simulink model "Final_System_Model_V10"  (R2018a)
settings: Solver=VariableStepAuto  StartTime=0  StopTime=250  FixedStep=0.5  RelTol=1e-3
PreLoadFcn:
  | Ts_Power=1e-6;
  | Ts_Control=100e-6;
undefined symbols (not defined in the file): DiscIntNeverNeededParam, sigbuilder_block
libraries: simulink x24, fl_lib x16, powerlib x15, nesl_utility x8, powerlib_meascontrol x5, re_lib x1
(part 6 of 8)

== system Final_System_Model_V10/Full System/Subsystem1/80KW Fuel Cell Stack_1/Load ==
  note: This Block models the Load Profile as dictated by the ship Resistance in the River Nile
  Signal : Inport
  Bus Selector : BusSelector  OutputSignals=Cell Output Voltage (V),Number Of Cells
  Current from Load profile of one day : Subsystem  Tag=STV Subsys  LoadFcn=sigbuilder_block('load');  StartFcn=sigbuilder_block('start');  StopFcn=sigbuilder_block('stop');  ClipboardFcn=sigbuilder_block('clipboard');  mask(Sigbuilder block){tuvar=[0:10]}
      mask help: Simulink:masks:SigbuilderBlock_MD
      mask init:
      | if ~strcmp(get_param(bdroot(gcbh),'SimulationStatus'),'stopped') tuvar = sigbuilder_block('maskInit'); end
      settings: CopyFcn=sigbuilder_block('copy');  DeleteFcn=sigbuilder_block('delete');  ModelCloseFcn=sigbuilder_block('modelClose');  PreSaveFcn=sigbuilder_block('preSave');  PauseFcn=sigbuilder_block('pause');  ContinueFcn=sigbuilder_block('continue');  NameChangeFcn=sigbuilder_block('namechange');  OpenFcn=sigbuilder_block('open',[403.5 117 550.5 359.25 ]);  CloseFcn=sigbuilder_block('close');
      mask Display: plot(0, 0, 100, 100,[2, 2, 32, 32, 2], [68, 8, 8, 68, 68],[32, 2], [38, 38], [32, 19, 2],[53, 60, 44], [32, 17, 17, 2],[16, 16, 31, 31]);txt = getActiveGroup(gcbh);text(2, 100, txt,'verticalAlignment', 'top');
  Product : Product
  Terminator : Terminator
  Terminator1 : Terminator
  Total Output Voltage (V) : Outport
  wires:
  Current from Load profile of one day/1(Signal 1) -> Terminator/1  "Current from Load profile (Alex to Aswan)"
  Bus Selector/2 -> Product/2  "<Number Of Cells>"
  Current from Load profile of one day/2(Signal 2) -> Terminator1/1  "Current from Load profile (Alex to Aswan)"
  Product/1 -> Total Output Voltage (V)/1  "Total Output Voltage (V)"
  Bus Selector/1 -> Product/1  "<Cell Output Voltage (V)>"
  Signal/1 -> Bus Selector/1

== system Final_System_Model_V10/Full System/Subsystem3/DC-DC converter1/Subsystem ==
  duty cycle : Inport
  I in : Inport  Port=2
  V in : Inport  Port=3
  Constant : Constant
  I out : Product  Inputs=*/
  Multiply : Product
  Multiply1 : Product
  Subtract : Sum  Inputs=+-
  V out : Product  Inputs=*/
  efficiency : Gain  Gain=0.98
  efficiency1 : Gain  Gain=0.98
  I o : Outport
  V o : Outport  Port=2
  wires:
  V in/1 -> efficiency1/1
  I out/1 -> I o/1
  V out/1 -> V o/1
  I in/1 -> efficiency/1
  efficiency1/1 -> Multiply1/1
  Multiply1/1 -> V out/1
  duty cycle/1 -> Multiply1/2, I out/2, Subtract/2
  Constant/1 -> Subtract/1
  Multiply/1 -> I out/1
  efficiency/1 -> Multiply/2
  Subtract/1 -> V out/2, Multiply/1

== system Final_System_Model_V10/Full System/Subsystem3/DC-DC converter1/duty cycle ==
  V in : Inport
  V req : Inport  Port=2
  Add : Sum
  Constant : Constant
  Divide : Product  Inputs=*/
  Gain : Gain  Gain=0.98
  Subtract : Sum  Inputs=+-
  tag scope: duty_cycle_battery=global
  wires:
  Divide/1 -> Subtract/2
  Gain/1 -> Add/1, Divide/1
  Add/1 -> Divide/2
  Constant/1 -> Subtract/1
  V in/1 -> Gain/1
  V req/1 -> Add/2
  Subtract/1 -> [duty_cycle_battery]

== system Final_System_Model_V10/Full System/Subsystem3/Subsystem/1st Mode ==
  delta : Inport
  Fuel Cells Output (KW) : Inport  Port=2
  Add : Sum  Inputs=+-
  Compare To Constant : simulink/Logic and Bit Operations/Compare To Constant  relop=>=  const=0  OutDataTypeStr=boolean
  Compare To Constant1 : simulink/Logic and Bit Operations/Compare To Constant  relop=<  const=72  OutDataTypeStr=boolean
  Logical Operator : Logic  AllPortsSameDT=off  OutDataTypeStr=boolean
  Switch15 : Switch  Criteria=u2 > Threshold
  Zero : Constant  Value=0
  Load to battery (KW) : Outport
  wires:
  Compare To Constant1/1 -> Logical Operator/2
  Compare To Constant/1 -> Logical Operator/1
  Zero/1 -> Switch15/3
  delta/1 -> Compare To Constant1/1, Add/1, Compare To Constant/1
  Switch15/1 -> Load to battery (KW)/1
  Logical Operator/1 -> Switch15/2
  Fuel Cells Output (KW)/1 -> Add/2
  Add/1 -> Switch15/1

== system Final_System_Model_V10/Full System/Subsystem3/Subsystem/2nd Mode ==
  delta : Inport
  Fuel Cells Output (KW) : Inport  Port=2
  Add : Sum  Inputs=+-
  Compare To Constant : simulink/Logic and Bit Operations/Compare To Constant  relop=>=  const=88  OutDataTypeStr=boolean
  Compare To Constant1 : simulink/Logic and Bit Operations/Compare To Constant  relop=<=  const=90  OutDataTypeStr=boolean
  Logical Operator : Logic  AllPortsSameDT=off  OutDataTypeStr=boolean
  Switch15 : Switch  Criteria=u2 > Threshold
  Zero : Constant  Value=0
  Battery to load (KW) : Outport
  wires:
  Switch15/1 -> Battery to load (KW)/1
  Fuel Cells Output (KW)/1 -> Add/2
  Compare To Constant1/1 -> Logical Operator/2
  Logical Operator/1 -> Switch15/2
  Compare To Constant/1 -> Logical Operator/1
  delta/1 -> Compare To Constant1/1, Compare To Constant/1, Add/1
  Zero/1 -> Switch15/3
  Add/1 -> Switch15/1

== system Final_System_Model_V10/Full System/Subsystem3/Subsystem/5th Mode ==
  delta : Inport
  Fuel Cells Output (KW) : Inport  Port=2
  Add : Sum  Inputs=+-
  Compare To Constant : simulink/Logic and Bit Operations/Compare To Constant  relop=>=  const=110  OutDataTypeStr=boolean
  Compare To Constant1 : simulink/Logic and Bit Operations/Compare To Constant  relop=<=  const=162  OutDataTypeStr=boolean
  Logical Operator : Logic  AllPortsSameDT=off  OutDataTypeStr=boolean
  Switch15 : Switch  Criteria=u2 > Threshold
  Zero : Constant  Value=0
  Battery to load (KW) : Outport
  wires:
  Add/1 -> Switch15/1
  Zero/1 -> Switch15/3
  delta/1 -> Add/1, Compare To Constant/1, Compare To Constant1/1
  Compare To Constant/1 -> Logical Operator/1
  Logical Operator/1 -> Switch15/2
  Compare To Constant1/1 -> Logical Operator/2
  Fuel Cells Output (KW)/1 -> Add/2
  Switch15/1 -> Battery to load (KW)/1

== system Final_System_Model_V10/Full System/Subsystem3/Subsystem/7th Mode ==
  delta : Inport
  Fuel Cells Output (KW) : Inport  Port=2
  Add : Sum  Inputs=+-
  Compare To Constant : simulink/Logic and Bit Operations/Compare To Constant  relop=>=  const=198  OutDataTypeStr=boolean
  Compare To Constant1 : simulink/Logic and Bit Operations/Compare To Constant  relop=<=  const=214  OutDataTypeStr=boolean
  Logical Operator : Logic  AllPortsSameDT=off  OutDataTypeStr=boolean
  Switch15 : Switch  Criteria=u2 > Threshold
  Zero : Constant  Value=0
  Battery to load (KW) : Outport
  wires:
  Switch15/1 -> Battery to load (KW)/1
  Fuel Cells Output (KW)/1 -> Add/2
  Compare To Constant1/1 -> Logical Operator/2
  Logical Operator/1 -> Switch15/2
  Compare To Constant/1 -> Logical Operator/1
  delta/1 -> Compare To Constant1/1, Compare To Constant/1, Add/1
  Zero/1 -> Switch15/3
  Add/1 -> Switch15/1

== system Final_System_Model_V10/Full System/Electrolysers/260 KW Electrolyzer Stack_1/electrolyser stack/electrolyser cell ==
  In1 : Inport
  In2 : Inport  Port=2
  In3 : Inport  Port=3
  (1/T)/(1/T_ref) : Subsystem
  Constant2 : Constant  Value=1/298
  Eta_B : Subsystem
  F : Constant  Value=96485.33289
  H2 flow rate : Subsystem
  R : Constant  Value=8.314
  Sum : Sum  Inputs=4
  V_0 : Subsystem
  eta_a : Subsystem
  eta_c : Subsystem
  Out1 : Outport
  Out2 : Outport  Port=2
  wires:
  eta_c/1(Out1) -> Sum/4
  In2/1 -> H2 flow rate/1(In1), eta_c/4(In4), eta_a/3(In3), Eta_B/3(In3)
  R/1 -> eta_a/2(In2), eta_a/4(In4), eta_c/2(In2), Eta_B/1(In1)
  In1/1 -> eta_a/5(In5), eta_c/3(In3), Eta_B/2(In2), (1/T)/(1/T_ref)/1(In1), V_0/1(In1)
  (1/T)/(1/T_ref)/1(Out1) -> eta_a/1(In1), eta_c/1(In1)
  eta_a/1(Out1) -> Sum/3
  Constant2/1 -> Eta_B/4(In4), (1/T)/(1/T_ref)/2(In2)
  Eta_B/1(Out1) -> Sum/2
  F/1 -> eta_a/6(In6), eta_c/5(In5), H2 flow rate/2(In2)
  V_0/1(Out1) -> Sum/1
  Sum/1 -> Out1/1
  In3/1 -> H2 flow rate/3(In3)
  H2 flow rate/1(Out1) -> Out2/1

== system Final_System_Model_V10/Full System/Electrolysers/93 KW Electrolyzer Stack_2/electrolyser stack/electrolyser cell ==
  In1 : Inport
  In2 : Inport  Port=2
  In3 : Inport  Port=3
  (1/T)/(1/T_ref) : Subsystem
  Constant2 : Constant  Value=1/298
  Eta_B : Subsystem
  F : Constant  Value=96485.33289
  H2 flow rate : Subsystem
  R : Constant  Value=8.314
  Sum : Sum  Inputs=4
  V_0 : Subsystem
  eta_a : Subsystem
  eta_c : Subsystem
  Out1 : Outport
  Out2 : Outport  Port=2
  wires:
  H2 flow rate/1(Out1) -> Out2/1
  In3/1 -> H2 flow rate/3(In3)
  Sum/1 -> Out1/1
  V_0/1(Out1) -> Sum/1
  F/1 -> H2 flow rate/2(In2), eta_c/5(In5), eta_a/6(In6)
  Eta_B/1(Out1) -> Sum/2
  Constant2/1 -> (1/T)/(1/T_ref)/2(In2), Eta_B/4(In4)
  eta_a/1(Out1) -> Sum/3
  (1/T)/(1/T_ref)/1(Out1) -> eta_c/1(In1), eta_a/1(In1)
  In1/1 -> V_0/1(In1), (1/T)/(1/T_ref)/1(In1), Eta_B/2(In2), eta_c/3(In3), eta_a/5(In5)
  R/1 -> Eta_B/1(In1), eta_c/2(In2), eta_a/4(In4), eta_a/2(In2)
  In2/1 -> Eta_B/3(In3), eta_a/3(In3), eta_c/4(In4), H2 flow rate/1(In1)
  eta_c/1(Out1) -> Sum/4

== system Final_System_Model_V10/Full System/Solar Panel + Solar Charge Controller/PV Insert inputs here/Subsystem/C to K Converter  ==
  T_o : Inport
  Sum : Sum  Inputs=|++
  Sum1 : Sum  Inputs=|++
  T_ref : Constant  Value=25
  constant : Constant  Value=273.12
  T_ak : Outport
  T_rk : Outport  Port=2
  wires:
  constant/1 -> Sum1/1, Sum/2
  T_o/1 -> Sum/1  "T_act (c)"
  T_ref/1 -> Sum1/2  "T_ref (c)"
  Sum/1 -> T_ak/1  "T_act(k)"
  Sum1/1 -> T_rk/1  "T_ref(k)"

== system Final_System_Model_V10/Full System/Solar Panel + Solar Charge Controller/PV Insert inputs here/Subsystem/I o ==
  T_ak : Inport
  T_rk : Inport  Port=2
  I_on : Inport  Port=3
  Constant : Constant
  Electron charge : Constant  Value=1.6*10^(-19)
  Exp(fn(1)) : Fcn  Expr=exp(u(1))
  Fcn : Fcn  Expr=(u(1))^3
  Product : Product  Inputs=/***/
  Product1 : Product  Inputs=*/
  Product2 : Product  Inputs=*/
  Product3 : Product  Inputs=*/
  Product4 : Product  Inputs=3
  Sum : Sum  Inputs=|+-
  band gap energy (Eg) : Constant  Value=1.1
  boltzamann constant : Constant  Value=1.3805*10^(-23)
  ideality factor depend on material : Constant  Value=1.14
  I_o : Outport
  wires:
  Electron charge/1 -> Product/2  "e"
  boltzamann constant/1 -> Product/1  "k"
  Product2/1 -> Sum/2  "1/T"
  I_on/1 -> Product4/3  "I_on"
  band gap energy (Eg)/1 -> Product/3  "Eg"
  Sum/1 -> Product/4  "((1/Tn)-(1/T))"
  Product3/1 -> Fcn/1  "T/Tn"
  Product1/1 -> Sum/1  "1/Tn"
  Constant/1 -> Product2/1, Product1/1
  ideality factor depend on material/1 -> Product/5  "a"
  T_ak/1 -> Product3/1, Product2/2
  Fcn/1 -> Product4/2  "(T/Tn)^3"
  Product/1 -> Exp(fn(1))/1  "Fn(1)"
  Exp(fn(1))/1 -> Product4/1  "Exp(fn(1))"
  T_rk/1 -> Product1/2, Product3/2
  Product4/1 -> I_o/1

== system Final_System_Model_V10/Full System/Solar Panel + Solar Charge Controller/PV Insert inputs here/Subsystem/I on ==
  T_ref : Inport
  I_scn : Inport  Port=2
  Num series : Inport  Port=3
  V_oc : Inport  Port=4
  Electron charge : Constant  Value=1.6*10^(-19)
  Fcn : Fcn  Expr=(u(1))/(exp(u(2))-u(1))
  Mux : Mux  Inputs=3
  Product : Product  Inputs=//**//
  boltzamann constant : Constant  Value=1.3805*10^(-23)
  constant : Constant
  ideality factor : Constant  Value=1.1415
  I_on : Outport
  wires:
  Num series/1 -> Product/1  "num_series_cells"
  boltzamann constant/1 -> Product/2  "K"
  Electron charge/1 -> Product/3  "q"
  ideality factor/1 -> Product/5  "a"
  T_ref/1 -> Product/6  "T_ref(k)"
  Product/1 -> Mux/2
  I_scn/1 -> Mux/1
  constant/1 -> Mux/3
  Mux/1 -> Fcn/1
  Fcn/1 -> I_on/1
  V_oc/1 -> Product/4

== system Final_System_Model_V10/Full System/Solar Panel + Solar Charge Controller/PV Insert inputs here/Subsystem/I ph due to radiation  ==
  insolation : Inport
  T_ak : Inport  Port=2
  T_rk : Inport  Port=3
  I_scn : Inport  Port=4
  Product : Product
  Product1 : Product
  SC_temp COFF const : Constant  Value=0.0017
  Sum : Sum  Inputs=|++
  Sum1 : Sum  Inputs=|+-
  I_photon : Outport
  wires:
  Product/1 -> I_photon/1  "photons current"
  insolation/1 -> Product/1
  T_ak/1 -> Sum1/1  "actual temp(k)"
  T_rk/1 -> Sum1/2  "referance temp(k)"
  Sum/1 -> Product/2
  I_scn/1 -> Sum/2  "nominal short circuit current"
  Product1/1 -> Sum/1
  SC_temp COFF const/1 -> Product1/1
  Sum1/1 -> Product1/2

== system Final_System_Model_V10/Full System/Solar Panel + Solar Charge Controller/PV Insert inputs here/Subsystem/I pv ==
  V_PV : Inport
  I_photon : Inport  Port=2
  I_o : Inport  Port=3
  Ns*A*Kt1 : Inport  Port=4
  Rp Shunt resistance : Inport  Port=5
  Electron charge : Constant  Value=1.6*10^(-19)
  IPV = u(3)-u(4)*(exp((u(2)*(u(1)+u(6)))/(u(5)))-1) : Fcn  Expr=u(3)-u(4)*(exp((u(2)*(u(1)+u(6)))/(u(5)))-1)-u(7)
  Mux : Mux  Inputs=7
  Product : Product  Inputs=*/
  Rs : Gain  Gain=.4
  Sum : Sum  Inputs=|++
  I_PV : Outport
  wires:
  IPV = u(3)-u(4)*(exp((u(2)*(u(1)+u(6)))/(u(5)))-1)/1 -> I_PV/1, Rs/1  "I_PV"
  Ns*A*Kt1/1 -> Mux/5
  Mux/1 -> IPV = u(3)-u(4)*(exp((u(2)*(u(1)+u(6)))/(u(5)))-1)/1
  I_o/1 -> Mux/4  "I_o"
  Rs/1 -> Sum/2, Mux/6  "I_PV*Rs"
  Electron charge/1 -> Mux/2  "q"
  I_photon/1 -> Mux/3  "I_ph"
  V_PV/1 -> Sum/1, Mux/1  "V_PV"
  Sum/1 -> Product/1
  Rp Shunt resistance/1 -> Product/2  "Shunt resistance"
  Product/1 -> Mux/7

== system Final_System_Model_V10/Full System/Solar Panel + Solar Charge Controller/PV Insert inputs here/Subsystem/NsAKt Thermal voltafe ==
  T_ak T in kelven : Inport
  N_series series cells : Constant  Value=96
  Product4 : Product  Inputs=4
  boltzamann constant : Constant  Value=1.3805*10^(-23)
  ideality factor depend on material : Constant  Value=1.17
  Ns*a*Kt : Outport
  wires:
  Product4/1 -> Ns*a*Kt/1
  boltzamann constant/1 -> Product4/2
  ideality factor depend on material/1 -> Product4/3
  T_ak T in kelven/1 -> Product4/1
  N_series series cells/1 -> Product4/4

== system Final_System_Model_V10/Full System/Solar Panel + Solar Charge Controller/Solar Charge Controller/MPPT Controller using  "Incremental Conductance + Integral Regulator "  technique /MPPT ==
  note: Maximum power point tracking by incremental conductance method
      | --------------------------------------------------------------
      | Maximum power point is obtained when dP/dV=0  where P= V*I
      | -> d(V*I)/dV = I + V*dI/dV = 0
      | -> dI/dV = -I/V
      |
      | dI, dV  = fundamental components of I and V ripples measured with a sliding time window T_MPPT
      | I , V   = mean values of V and I measured with a sliding time window T_MPPT
      |
      | The integral regulator minimizes the error (dI/dV + I/V)
      | Regulator output = Duty cycle correction
  V_PV : Inport
  I_PV : Inport  Port=2
  on/off : Inport  Port=3
  Add : Sum  Inputs=+-
  Add1 : Sum
  Constant : Constant  Value=0
  Constant1 : Constant  Value=0
  Dead Zone : DeadZone  LowerValue=-0.05  UpperValue=0.05  SaturateOnIntegerOverflow=on
  Discrete-Time Integrator : DiscreteIntegrator  SampleTime=Ts_Control  LimitOutput=on  UpperSaturationLimit=1  LowerSaturationLimit=-1  ICPrevOutput=DiscIntNeverNeededParam  ICPrevScaledInput=DiscIntNeverNeededParam
  Fourier : powerlib_meascontrol/Measurements/Fourier  Freq=1/T_MPPT  n=1  InInit=[0, 0]  Ts=Ts_Control
      settings: SourceProductName=Simscape Power Systems
  Fourier1 : powerlib_meascontrol/Measurements/Fourier  Freq=1/T_MPPT  n=1  InInit=[0, 0]  Ts=Ts_Control
      settings: SourceProductName=Simscape Power Systems
  MPPT Gain : Gain  Gain=5
  Mean : powerlib_meascontrol/Measurements/Mean  Freq=1/T_MPPT  Vinit=0  Ts=Ts_Control
  Mean1 : powerlib_meascontrol/Measurements/Mean  Freq=1/T_MPPT  Vinit=0  Ts=Ts_Control
  Saturation : Saturate  UpperLimit=inf  LowerLimit=eps
  Saturation1 : Saturate  UpperLimit=inf  LowerLimit=eps
  Switch : Switch  Threshold=0.5
  Switch1 : Switch  Threshold=0.5
  Trigonometric Function : Trigonometry  Operator=cos
  deg2rad : Gain  Gain=pi/180
  div : Product  Inputs=*/  RndMeth=Zero
  div1 : Product  Inputs=**  RndMeth=Zero
  div2 : Product  Inputs=*/  RndMeth=Zero
  Delta_D : Outport
  wires:
  Dead Zone/1 -> MPPT Gain/1
  Switch/1 -> Dead Zone/1  "error"
  Saturation1/1 -> div/2
  Saturation/1 -> div2/2
  Switch1/1 -> Delta_D/1
  on/off/1 -> Switch/2, Switch1/2
  Constant1/1 -> Switch1/3
  Discrete-Time Integrator/1 -> Switch1/1  "Delta_D"
  Constant/1 -> Switch/3
  MPPT Gain/1 -> Discrete-Time Integrator/1
  Add1/1 -> Switch/1  "error"
  div2/1 -> Add1/2  "I/V"
  Mean1/1 -> Saturation/1
  Mean/1 -> div2/1
  div1/1 -> Add1/1  "dI/dV"
  Trigonometric Function/1 -> div1/2
  div/1 -> div1/1
  deg2rad/1 -> Trigonometric Function/1
  Add/1 -> deg2rad/1
  Fourier1/1 -> Saturation1/1
  Fourier1/2 -> Add/2
  Fourier/2 -> Add/1
  V_PV/1 -> Mean1/1, Fourier1/1
  I_PV/1 -> Mean/1, Fourier/1
  Fourier/1 -> div/1

== system Final_System_Model_V10/Full System/Solar Panel + Solar Charge Controller/Solar Charge Controller MPPT it is a device which track a point which has the max power/MPPT /P&O  ==
  I_pv : Inport
  V_PV : Inport  Port=2
  P & O : Subsystem
  Saturation : Saturate  UpperLimit=1
  Subsystem1 : Subsystem
  Signal : Outport
  wires:
  P & O/1(signal) -> Saturation/1
  V_PV/1 -> P & O/2(Vpv)
  Saturation/1 -> Subsystem1/1(In1)
  Subsystem1/1(Out1) -> Signal/1
  I_pv/1 -> P & O/1(Ipv)

== system Final_System_Model_V10/Full System/Subsystem1/100KW Fuel Cell Stack_2/From Load Current and Fuel Cell Output Current (A) to Valve Restriction Area (m^2)/Subsystem ==
  In1 : Inport
  Add1 : Sum  Inputs=4
  Bus Creator1 : BusCreator  Inputs=7
  Bus Selector1 : BusSelector  OutputSignals=Output Current (A),3,3:0735e-14,Output Current (A),2,-5:0428e-11,Output Current (A),4:1772e-08,2:7105e-07
  Constant10 : Constant  Value=4.1772e-08
  Constant11 : Constant  Value=2.7105e-07
  Constant6 : Constant  Value=3
  Constant7 : Constant  Value=3.0735e-14
  Constant8 : Constant  Value=2
  Constant9 : Constant  Value=-5.0428e-11
  Math Function2 : Math  Operator=pow  SaturateOnIntegerOverflow=on
  Math Function3 : Math  Operator=pow  SaturateOnIntegerOverflow=on
  Product3 : Product
  Product4 : Product
  Product5 : Product
  Unit Delay3 : UnitDelay  SampleTime=-1
  Valve Opening from Output Current : Outport
  wires:
  Product3/1 -> Add1/1
  Constant9/1 -> Bus Creator1/5  "-5:0428e-11"
  Constant11/1 -> Bus Creator1/7  "2:7105e-07"
  Constant8/1 -> Bus Creator1/4  "2"
  Constant6/1 -> Bus Creator1/2  "3"
  Bus Selector1/5 -> Math Function3/2  "<2>"
  Constant10/1 -> Bus Creator1/6  "4:1772e-08"
  In1/1 -> Unit Delay3/1
  Math Function2/1 -> Product3/1
  Math Function3/1 -> Product4/1
  Bus Selector1/3 -> Product3/2  "<3:0735e-14>"
  Bus Selector1/9 -> Add1/4  "<2:7105e-07>"
  Bus Selector1/2 -> Math Function2/2  "<3>"
  Bus Creator1/1 -> Bus Selector1/1
  Bus Selector1/6 -> Product4/2  "<-5:0428e-11>"
  Bus Selector1/8 -> Product5/2  "<4:1772e-08>"
  Bus Selector1/4 -> Math Function3/1  "<Output Current (A)>"
  Product4/1 -> Add1/2
  Product5/1 -> Add1/3
  Constant7/1 -> Bus Creator1/3  "3:0735e-14"
  Unit Delay3/1 -> Bus Creator1/1  "Output Current (A)"
  Bus Selector1/7 -> Product5/1  "<Output Current (A)>"
  Bus Selector1/1 -> Math Function2/1  "<Output Current (A)>"
  Add1/1 -> Valve Opening from Output Current/1  "Valve Opening from Output Current"

== system Final_System_Model_V10/Full System/Subsystem1/100KW Fuel Cell Stack_2/From Load Current and Fuel Cell Output Current (A) to Valve Restriction Area (m^2)/Subsystem1 ==
  In1 : Inport
  Add : Sum  Inputs=4
  Bus Creator : BusCreator  Inputs=7
  Bus Selector : BusSelector  OutputSignals=|
      | Load Profile Current (A).Required Current
      | (A),3,3:0735e-14,Load Profile Current (A).Required Current
      | (A),2,-5:0428e-11,Load Profile Current (A).Required Current
      | (A),4:1772e-08,2:7105e-07
  Constant : Constant  Value=3
  Constant1 : Constant  Value=3.0735e-14
  Constant2 : Constant  Value=2
  Constant3 : Constant  Value=-5.0428e-11
  Constant4 : Constant  Value=4.1772e-08
  Constant5 : Constant  Value=2.7105e-07
  Math Function : Math  Operator=pow  SaturateOnIntegerOverflow=on
  Math Function1 : Math  Operator=pow  SaturateOnIntegerOverflow=on
  Product : Product
  Product1 : Product
  Product2 : Product
  Unit Delay2 : UnitDelay  SampleTime=-1
  Out1 : Outport
  wires:
  Bus Selector/2 -> Math Function/2  "<3>"
  Bus Selector/5 -> Math Function1/2  "<2>"
  Product/1 -> Add/1
  Constant/1 -> Bus Creator/2  "3"
  Unit Delay2/1 -> Bus Creator/1  "Load Profile Current (A)"
  Constant5/1 -> Bus Creator/7  "2:7105e-07"
  Constant2/1 -> Bus Creator/4  "2"
  Bus Selector/1 -> Math Function/1  "<Required Current (A)>"
  Constant3/1 -> Bus Creator/5  "-5:0428e-11"
  Constant4/1 -> Bus Creator/6  "4:1772e-08"
  Bus Selector/7 -> Product2/1  "<Required Current (A)>"
  Math Function1/1 -> Product1/1
  Bus Selector/9 -> Add/4  "<2:7105e-07>"
  Bus Selector/8 -> Product2/2  "<4:1772e-08>"
  Bus Selector/6 -> Product1/2  "<-5:0428e-11>"
  Constant1/1 -> Bus Creator/3  "3:0735e-14"
  Product1/1 -> Add/2
  Math Function/1 -> Product/1
  Bus Creator/1 -> Bus Selector/1
  Product2/1 -> Add/3
  Bus Selector/3 -> Product/2  "<3:0735e-14>"
  Bus Selector/4 -> Math Function1/1  "<Required Current (A)>"
  In1/1 -> Unit Delay2/1
  Add/1 -> Out1/1

== system Final_System_Model_V10/Full System/Subsystem1/100KW Fuel Cell Stack_2/Fuel Cell Model/ From Current Density (A//cm^2) To Overvoltages (V) ==
  note: This Block calculates all the Resistances in the Fuel Cell
      | 1-Activation Overvoltage 2- Ohmic Overvoltage 3-Concentration Overvoltage
      | INPUTS: INPUTS: A) Current Density (A/cm^2) INPUTS: A) Current Density (A/cm^2)
      | A) Current Density (A/cm^2) OUTPUTS: A) Ohmic Overvoltage (V) OUTPUTS: A) Concentration Overvoltage (V)
      | B) Temperature (c)
      |
      | OUTPUTS:
      | A) Activation Overvoltage (V)
  Current Density (A/cm^2) : Inport
  Temperature (C) : Inport  Port=2
  Activation Overvoltage : Subsystem
  Concentration Overvoltage : Subsystem
  Ohmic Overvoltage : Subsystem
  Activation Overvoltage (V) : Outport
  Ohmic Overvoltage (V) : Outport  Port=2
  Concentration Overvoltage (V) : Outport  Port=3
  Exchange Current Density (i_0) : Outport  Port=4
  wires:
  Temperature (C)/1 -> Activation Overvoltage/1(Temperature/C1)
  Current Density (A/cm^2)/1 -> Activation Overvoltage/2(Current Density (i)(A/cm^2)), Concentration Overvoltage/1(Current Density (i)1), Ohmic Overvoltage/1(Current Density (i ))
  Ohmic Overvoltage/1(V_Resistive) -> Ohmic Overvoltage (V)/1
  Activation Overvoltage/1(Activation Overvoltage1 (V)) -> Activation Overvoltage (V)/1
  Concentration Overvoltage/1("Concentration Overvoltage1 (V) ") -> Concentration Overvoltage (V)/1
  Activation Overvoltage/2(Exchange Current Density (i_0)) -> Exchange Current Density (i_0)/1

== system Final_System_Model_V10/Full System/Subsystem1/100KW Fuel Cell Stack_2/Fuel Cell Model/Air Flow Rate To Current (A) ==
  note: The function of this block is: To calculate the Air Mass Flow Rate in (kg/s) using the Input Current Density (A/cm^2)
      | Inputs: Outputs:
      | a) Current DEnsity (A/cm^2) A) Air Mass Flow Rate (kg/s)
      | b) Cell Area (cm^2)
      | c) Number of Cells
  Current Density (A/cm^2) : Inport
  Cell Area (cm^2) : Inport  Port=2
  Number Of Cells : Inport  Port=3
  Air Molar Mass (Kg) : Constant  Value=28.9647e-3
  Current (A) : Product
  Divide : Product  Inputs=*/
  From Stack Current (A) To Oxygen Mass Flow Rate(kg/s) : Subsystem
  Oxygen Molar Mass per One Mole of Air (Kg) : Constant  Value=6.72e-3
  Product : Product
  Air Mass Flow Rate (kg/s) : Outport
  wires:
  Current (A)/1 -> From Stack Current (A) To Oxygen Mass Flow Rate(kg/s)/1(Current (A))
  Number Of Cells/1 -> From Stack Current (A) To Oxygen Mass Flow Rate(kg/s)/2(Number Of Cells)
  From Stack Current (A) To Oxygen Mass Flow Rate(kg/s)/1(Oxygen Flow Rate (kg/s)) -> Product/1
  Current Density (A/cm^2)/1 -> Current (A)/1
  Cell Area (cm^2)/1 -> Current (A)/2
  Air Molar Mass (Kg)/1 -> Product/2
  Product/1 -> Divide/1
  Oxygen Molar Mass per One Mole of Air (Kg)/1 -> Divide/2
  Divide/1 -> Air Mass Flow Rate (kg/s)/1  "Air Mass Flow Rate (kg/s)"

== system Final_System_Model_V10/Full System/Subsystem1/100KW Fuel Cell Stack_2/Fuel Cell Model/Current Density A//cm^2 (Polarization Curve) ==
  Demux : Demux  Tag=STV Demux  Outputs=2
  FromWs : FromWorkspace  Tag=STV FromWs  VariableName=tuvar  SampleTime=0
      SigBuilderData=|
      | common.afterFinalStr = 'Extrapolate'
      | common.sampleTime = 0
      | dataSet.timeRange = [0 20]
      | dataSet.name = 'Group 1'
      | sbobj.Groups.Name = 'Group 1'
      | sbobj.Groups.Signals(1).Name = 'Signal 1'
      | sbobj.Groups.Signals(1).XData = [0 0.5 1 20]
      | sbobj.Groups.Signals(1).YData = [0.01 1 1.4 1.4]
      | sbobj.Groups.Signals(2).Name = 'Signal 2'
      | sbobj.Groups.Signals(2).XData = [0 20]
      | sbobj.Groups.Signals(2).YData = [1 1]
      | sbobj.Groups.TimeRange = [0 20]
  Signal 1 : Outport  Tag=STV Outport
  Signal 2 : Outport  Tag=STV Outport  Port=2
  wires:
  Demux/1 -> Signal 1/1
  FromWs/1 -> Demux/1
  Demux/2 -> Signal 2/1

== system Final_System_Model_V10/Full System/Subsystem1/100KW Fuel Cell Stack_2/Fuel Cell Model/From Mass Flow Rates (kg//s) To Current Density (A//cm^2) ==
  note: The function of this block is to convert the input Hydrogen Mass Flow rate (Kg/s) to Current (A) then divide it by the Cell Area (cm^2) to get (Current Density) (A/cm^2)
      | which will be the input of several other blocks.
      | Inputs: a)Hydrogen Mass Flow Rate (kg/s) Outputs: Current Density (A/cm^2)
      | b)Number of Cells
      | c) Cell Area (cm^2)
  Hydrogen Flow Rate (kg/s) : Inport
  Cell Area (cm^2) : Inport  Port=2
  Number Of Cells : Inport  Port=3
  From Current (A) To Current Density (A/cm^2) : Subsystem
  Fuel Mass Flow Rate (kg/s) To Current (A) : Subsystem
  Current Density (A/cm^2) : Outport
  wires:
  Cell Area (cm^2)/1 -> From Current (A) To Current Density (A/cm^2)/2(Cell Area (cm^2))
  Fuel Mass Flow Rate (kg/s) To Current (A)/1(Current (A)) -> From Current (A) To Current Density (A/cm^2)/1(Nominal Current (A))
  Hydrogen Flow Rate (kg/s)/1 -> Fuel Mass Flow Rate (kg/s) To Current (A)/1(Hydrogen Flow Rate (kg/s))
  From Current (A) To Current Density (A/cm^2)/1(Current Density (A/cm^2)) -> Current Density (A/cm^2)/1  "Current density (A/cm^2)"
  Number Of Cells/1 -> Fuel Mass Flow Rate (kg/s) To Current (A)/2(Number Of Cells)  "Number Of Cells"

== system Final_System_Model_V10/Full System/Subsystem1/100KW Fuel Cell Stack_2/Fuel Cell Model/From Pressures (atm) To Nernest Voltage (V) ==
  note: This Block calculates the Partial Pressures of Hydrogen and Oxygen (atm) from their pressures (atm) then uses these values to calculate the Nernest Voltage (V)
      |
      | INPUTS: A) Current Density (i) (A/cm^2) OUTPUTS 1: A) Oxygen Partial Pressure (atm) OUTPUTS 2: A) Nernest Voltage (V)
      | B) Absolute Hydrogen Pressure (atm) B) Water Saturation Pressure (atm)
      | C) Absolute Air Pressure (atm) C) Hydrogen Partial Pressure(atm)
      | D) Temperature (c)
  Current Density (i) : Inport
  Hydrogen Pressure (atm) : Inport  Port=2
  Air Pressure (atm) : Inport  Port=3
  Temperature (C) : Inport  Port=4
  From Absolute Pressure (atm) To Partial Pressures (atm) : Subsystem
  From Partial Pressures (atm) To Nernest Voltage (V) : Subsystem
  Oxygen Partial Pressure : Outport
  Nernest Voltage (V) : Outport  Port=2
  Water Pressure : Outport  Port=3
  wires:
  Temperature (C)/1 -> From Partial Pressures (atm) To Nernest Voltage (V)/4(Temperature/C), From Absolute Pressure (atm) To Partial Pressures (atm)/4(Temperature/C)
  From Absolute Pressure (atm) To Partial Pressures (atm)/1(Hydrogen Partial Pressure (pp_H2)) -> From Partial Pressures (atm) To Nernest Voltage (V)/1(Hydrogen Partial Pressure)
  Hydrogen Pressure (atm)/1 -> From Absolute Pressure (atm) To Partial Pressures (atm)/2(Hydrogen Pressure (P_H2))
  From Partial Pressures (atm) To Nernest Voltage (V)/1(Nernest Voltage1) -> Nernest Voltage (V)/1
  From Absolute Pressure (atm) To Partial Pressures (atm)/2(Oxygen Partial Pressure pp_O2) -> Oxygen Partial Pressure/1, From Partial Pressures (atm) To Nernest Voltage (V)/2(Oxygen Partial Pressure)
  From Absolute Pressure (atm) To Partial Pressures (atm)/3(Water Pressure) -> Water Pressure/1, From Partial Pressures (atm) To Nernest Voltage (V)/3(Water Pressure (P_H2O))
  Current Density (i)/1 -> From Absolute Pressure (atm) To Partial Pressures (atm)/1(Current Density (i ))
  Air Pressure (atm)/1 -> From Absolute Pressure (atm) To Partial Pressures (atm)/3(Air Pressure (P_air))

== system Final_System_Model_V10/Full System/Subsystem1/100KW Fuel Cell Stack_2/Load/Current from Load profile of one day ==
  Demux : Demux  Tag=STV Demux  Outputs=2
  FromWs : FromWorkspace  Tag=STV FromWs  VariableName=tuvar  SampleTime=0
      SigBuilderData=|
      | common.afterFinalStr = 'Extrapolate'
      | common.sampleTime = 0
      | dataSet.timeRange = [0 300]
      | dataSet.name = 'Group 1'
      | sbobj.Groups.Name = 'Group 1'
      | sbobj.Groups.Signals(1).Name = 'Signal 1'
      | sbobj.Groups.Signals(1).XData = [0 2.75 2.75 5.75 5.75 10.98 10.98 24 24 24.6 24.6 27.61 27.61 30.61 30.61 33.73 33.73 36.73 48 48 52.19 52.19 55.19 55.19 59.38 59.38 62.38 72 72 84 84 96 96 108 108 120 120 132 132 144 144 146.76 146.76 147.76 147.76 156 156 168 168 175.76 175.76 176.76 176.76 180 180 192 192 204 204 216 216 216.76 216.76 217.76 217.76 228 228 240 240 244.83 244.83 300]
      | sbobj.Groups.Signals(1).YData = [145.4545455 145.4545455 0.01 0.01 145.4545455 145.4545455 0.01 0.01 195.4545455 195.4545455 486.3636364 486.3636364 0.01 0.01 404.5454545 404.5454545 0.01 0.01 0.01 486.3636364 486.3636364 0.01 0.01 486.3636364 486.3636364 0.01 0.01 0.01 463.6363636 463.6363636 0.01 0.01 463.6363636 463.6363636 0.01 0.01 463.6363636 463.6363636 0.01 0.01 463.6363636 463.6363636 0.01 0.01 463.6363636 463.6363636 0.01 0.01 463.6363636 463.6363636 0.01 0.01 463.6363636 463.6363636 0.01 0.01 463.6363636 463.6363636 0.01 0.01 463.6363636 463.6363636 0.01 0.01 463.6363636 463.6363636 0.01 0.01 463.6363636 463.6363636 0.01 0.01]
      | sbobj.Groups.Signals(2).Name = 'Signal 2'
      | sbobj.Groups.Signals(2).XData = [0 300]
      | sbobj.Groups.Signals(2).YData = [243 243]
      | sbobj.Groups.TimeRange = [0 300]
  Signal 1 : Outport  Tag=STV Outport
  Signal 2 : Outport  Tag=STV Outport  Port=2
  wires:
  Demux/1 -> Signal 1/1
  FromWs/1 -> Demux/1
  Demux/2 -> Signal 2/1

== system Final_System_Model_V10/Full System/Subsystem1/80KW Fuel Cell Stack_1/From Load Current and Fuel Cell Output Current (A) to Valve Restriction Area (m^2)/Subsystem ==
  In1 : Inport
  Add1 : Sum  Inputs=4
  Bus Creator1 : BusCreator  Inputs=7
  Bus Selector1 : BusSelector  OutputSignals=Output Current (A),3,3:0735e-14,Output Current (A),2,-5:0428e-11,Output Current (A),4:1772e-08,2:7105e-07
  Constant10 : Constant  Value=4.1772e-08
  Constant11 : Constant  Value=2.7105e-07
  Constant6 : Constant  Value=3
  Constant7 : Constant  Value=3.0735e-14
  Constant8 : Constant  Value=2
  Constant9 : Constant  Value=-5.0428e-11
  Math Function2 : Math  Operator=pow  SaturateOnIntegerOverflow=on
  Math Function3 : Math  Operator=pow  SaturateOnIntegerOverflow=on
  Product3 : Product
  Product4 : Product
  Product5 : Product
  Unit Delay3 : UnitDelay  SampleTime=-1
  Valve Opening from Output Current : Outport
  wires:
  Add1/1 -> Valve Opening from Output Current/1  "Valve Opening from Output Current"
  Bus Selector1/1 -> Math Function2/1  "<Output Current (A)>"
  Bus Selector1/7 -> Product5/1  "<Output Current (A)>"
  Unit Delay3/1 -> Bus Creator1/1  "Output Current (A)"
  Constant7/1 -> Bus Creator1/3  "3:0735e-14"
  Product5/1 -> Add1/3
  Product4/1 -> Add1/2
  Bus Selector1/4 -> Math Function3/1  "<Output Current (A)>"
  Bus Selector1/8 -> Product5/2  "<4:1772e-08>"
  Bus Selector1/6 -> Product4/2  "<-5:0428e-11>"
  Bus Creator1/1 -> Bus Selector1/1
  Bus Selector1/2 -> Math Function2/2  "<3>"
  Bus Selector1/9 -> Add1/4  "<2:7105e-07>"
  Bus Selector1/3 -> Product3/2  "<3:0735e-14>"
  Math Function3/1 -> Product4/1
  Math Function2/1 -> Product3/1
  In1/1 -> Unit Delay3/1
  Constant10/1 -> Bus Creator1/6  "4:1772e-08"
  Bus Selector1/5 -> Math Function3/2  "<2>"
  Constant6/1 -> Bus Creator1/2  "3"
  Constant8/1 -> Bus Creator1/4  "2"
  Constant11/1 -> Bus Creator1/7  "2:7105e-07"
  Constant9/1 -> Bus Creator1/5  "-5:0428e-11"
  Product3/1 -> Add1/1

== system Final_System_Model_V10/Full System/Subsystem1/80KW Fuel Cell Stack_1/From Load Current and Fuel Cell Output Current (A) to Valve Restriction Area (m^2)/Subsystem1 ==
  In1 : Inport
  Add : Sum  Inputs=4
  Bus Creator : BusCreator  Inputs=7
  Bus Selector : BusSelector  OutputSignals=|
      | Load Profile Current (A).Required Current
      | (A),3,3:0735e-14,Load Profile Current (A).Required Current
      | (A),2,-5:0428e-11,Load Profile Current (A).Required Current
      | (A),4:1772e-08,2:7105e-07
  Constant : Constant  Value=3
  Constant1 : Constant  Value=3.0735e-14
  Constant2 : Constant  Value=2
  Constant3 : Constant  Value=-5.0428e-11
  Constant4 : Constant  Value=4.1772e-08
  Constant5 : Constant  Value=2.7105e-07
  Math Function : Math  Operator=pow  SaturateOnIntegerOverflow=on
  Math Function1 : Math  Operator=pow  SaturateOnIntegerOverflow=on
  Product : Product
  Product1 : Product
  Product2 : Product
  Unit Delay2 : UnitDelay  SampleTime=-1
  Out1 : Outport
  wires:
  Add/1 -> Out1/1
  In1/1 -> Unit Delay2/1
  Bus Selector/4 -> Math Function1/1  "<Required Current (A)>"
  Bus Selector/3 -> Product/2  "<3:0735e-14>"
  Product2/1 -> Add/3
  Bus Creator/1 -> Bus Selector/1
  Math Function/1 -> Product/1
  Product1/1 -> Add/2
  Constant1/1 -> Bus Creator/3  "3:0735e-14"
  Bus Selector/6 -> Product1/2  "<-5:0428e-11>"
  Bus Selector/8 -> Product2/2  "<4:1772e-08>"
  Bus Selector/9 -> Add/4  "<2:7105e-07>"
  Math Function1/1 -> Product1/1
  Bus Selector/7 -> Product2/1  "<Required Current (A)>"
  Constant4/1 -> Bus Creator/6  "4:1772e-08"
  Constant3/1 -> Bus Creator/5  "-5:0428e-11"
  Bus Selector/1 -> Math Function/1  "<Required Current (A)>"
  Constant2/1 -> Bus Creator/4  "2"
  Constant5/1 -> Bus Creator/7  "2:7105e-07"
  Unit Delay2/1 -> Bus Creator/1  "Load Profile Current (A)"
  Constant/1 -> Bus Creator/2  "3"
  Product/1 -> Add/1
  Bus Selector/5 -> Math Function1/2  "<2>"
  Bus Selector/2 -> Math Function/2  "<3>"

== system Final_System_Model_V10/Full System/Subsystem1/80KW Fuel Cell Stack_1/Fuel Cell Model/ From Current Density (A//cm^2) To Overvoltages (V) ==
  note: This Block calculates all the Resistances in the Fuel Cell
      | 1-Activation Overvoltage 2- Ohmic Overvoltage 3-Concentration Overvoltage
      | INPUTS: INPUTS: A) Current Density (A/cm^2) INPUTS: A) Current Density (A/cm^2)
      | A) Current Density (A/cm^2) OUTPUTS: A) Ohmic Overvoltage (V) OUTPUTS: A) Concentration Overvoltage (V)
      | B) Temperature (c)
      |
      | OUTPUTS:
      | A) Activation Overvoltage (V)
  Current Density (A/cm^2) : Inport
  Temperature (C) : Inport  Port=2
  Activation Overvoltage : Subsystem
  Concentration Overvoltage : Subsystem
  Ohmic Overvoltage : Subsystem
  Activation Overvoltage (V) : Outport
  Ohmic Overvoltage (V) : Outport  Port=2
  Concentration Overvoltage (V) : Outport  Port=3
  Exchange Current Density (i_0) : Outport  Port=4
  wires:
  Activation Overvoltage/2(Exchange Current Density (i_0)) -> Exchange Current Density (i_0)/1
  Concentration Overvoltage/1("Concentration Overvoltage1 (V) ") -> Concentration Overvoltage (V)/1
  Activation Overvoltage/1(Activation Overvoltage1 (V)) -> Activation Overvoltage (V)/1
  Ohmic Overvoltage/1(V_Resistive) -> Ohmic Overvoltage (V)/1
  Current Density (A/cm^2)/1 -> Ohmic Overvoltage/1(Current Density (i )), Concentration Overvoltage/1(Current Density (i)1), Activation Overvoltage/2(Current Density (i)(A/cm^2))
  Temperature (C)/1 -> Activation Overvoltage/1(Temperature/C1)

== system Final_System_Model_V10/Full System/Subsystem1/80KW Fuel Cell Stack_1/Fuel Cell Model/Air Flow Rate To Current (A) ==
  note: The function of this block is: To calculate the Air Mass Flow Rate in (kg/s) using the Input Current Density (A/cm^2)
      | Inputs: Outputs:
      | a) Current DEnsity (A/cm^2) A) Air Mass Flow Rate (kg/s)
      | b) Cell Area (cm^2)
      | c) Number of Cells
  Current Density (A/cm^2) : Inport
  Cell Area (cm^2) : Inport  Port=2
  Number Of Cells : Inport  Port=3
  Air Molar Mass (Kg) : Constant  Value=28.9647e-3
  Current (A) : Product
  Divide : Product  Inputs=*/
  From Stack Current (A) To Oxygen Mass Flow Rate(kg/s) : Subsystem
  Oxygen Molar Mass per One Mole of Air (Kg) : Constant  Value=6.72e-3
  Product : Product
  Air Mass Flow Rate (kg/s) : Outport
  wires:
  Divide/1 -> Air Mass Flow Rate (kg/s)/1  "Air Mass Flow Rate (kg/s)"
  Oxygen Molar Mass per One Mole of Air (Kg)/1 -> Divide/2
  Product/1 -> Divide/1
  Air Molar Mass (Kg)/1 -> Product/2
  Cell Area (cm^2)/1 -> Current (A)/2
  Current Density (A/cm^2)/1 -> Current (A)/1
  From Stack Current (A) To Oxygen Mass Flow Rate(kg/s)/1(Oxygen Flow Rate (kg/s)) -> Product/1
  Number Of Cells/1 -> From Stack Current (A) To Oxygen Mass Flow Rate(kg/s)/2(Number Of Cells)
  Current (A)/1 -> From Stack Current (A) To Oxygen Mass Flow Rate(kg/s)/1(Current (A))

== system Final_System_Model_V10/Full System/Subsystem1/80KW Fuel Cell Stack_1/Fuel Cell Model/Current Density A//cm^2 (Polarization Curve) ==
  Demux : Demux  Tag=STV Demux  Outputs=2
  FromWs : FromWorkspace  Tag=STV FromWs  VariableName=tuvar  SampleTime=0
      SigBuilderData=|
      | common.afterFinalStr = 'Extrapolate'
      | common.sampleTime = 0
      | dataSet.timeRange = [0 20]
      | dataSet.name = 'Group 1'
      | sbobj.Groups.Name = 'Group 1'
      | sbobj.Groups.Signals(1).Name = 'Signal 1'
      | sbobj.Groups.Signals(1).XData = [0 0.5 1 20]
      | sbobj.Groups.Signals(1).YData = [0.01 1 1.4 1.4]
      | sbobj.Groups.Signals(2).Name = 'Signal 2'
      | sbobj.Groups.Signals(2).XData = [0 20]
      | sbobj.Groups.Signals(2).YData = [1 1]
      | sbobj.Groups.TimeRange = [0 20]
  Signal 1 : Outport  Tag=STV Outport
  Signal 2 : Outport  Tag=STV Outport  Port=2
  wires:
  Demux/2 -> Signal 2/1
  FromWs/1 -> Demux/1
  Demux/1 -> Signal 1/1

== system Final_System_Model_V10/Full System/Subsystem1/80KW Fuel Cell Stack_1/Fuel Cell Model/From Mass Flow Rates (kg//s) To Current Density (A//cm^2) ==
  note: The function of this block is to convert the input Hydrogen Mass Flow rate (Kg/s) to Current (A) then divide it by the Cell Area (cm^2) to get (Current Density) (A/cm^2)
      | which will be the input of several other blocks.
      | Inputs: a)Hydrogen Mass Flow Rate (kg/s) Outputs: Current Density (A/cm^2)
      | b)Number of Cells
      | c) Cell Area (cm^2)
  Hydrogen Flow Rate (kg/s) : Inport
  Cell Area (cm^2) : Inport  Port=2
  Number Of Cells : Inport  Port=3
  From Current (A) To Current Density (A/cm^2) : Subsystem
  Fuel Mass Flow Rate (kg/s) To Current (A) : Subsystem
  Current Density (A/cm^2) : Outport
  wires:
  Number Of Cells/1 -> Fuel Mass Flow Rate (kg/s) To Current (A)/2(Number Of Cells)  "Number Of Cells"
  From Current (A) To Current Density (A/cm^2)/1(Current Density (A/cm^2)) -> Current Density (A/cm^2)/1  "Current density (A/cm^2)"
  Hydrogen Flow Rate (kg/s)/1 -> Fuel Mass Flow Rate (kg/s) To Current (A)/1(Hydrogen Flow Rate (kg/s))
  Fuel Mass Flow Rate (kg/s) To Current (A)/1(Current (A)) -> From Current (A) To Current Density (A/cm^2)/1(Nominal Current (A))
  Cell Area (cm^2)/1 -> From Current (A) To Current Density (A/cm^2)/2(Cell Area (cm^2))

== system Final_System_Model_V10/Full System/Subsystem1/80KW Fuel Cell Stack_1/Fuel Cell Model/From Pressures (atm) To Nernest Voltage (V) ==
  note: This Block calculates the Partial Pressures of Hydrogen and Oxygen (atm) from their pressures (atm) then uses these values to calculate the Nernest Voltage (V)
      |
      | INPUTS: A) Current Density (i) (A/cm^2) OUTPUTS 1: A) Oxygen Partial Pressure (atm) OUTPUTS 2: A) Nernest Voltage (V)
      | B) Absolute Hydrogen Pressure (atm) B) Water Saturation Pressure (atm)
      | C) Absolute Air Pressure (atm) C) Hydrogen Partial Pressure(atm)
      | D) Temperature (c)
  Current Density (i) : Inport
  Hydrogen Pressure (atm) : Inport  Port=2
  Air Pressure (atm) : Inport  Port=3
  Temperature (C) : Inport  Port=4
  From Absolute Pressure (atm) To Partial Pressures (atm) : Subsystem
  From Partial Pressures (atm) To Nernest Voltage (V) : Subsystem
  Oxygen Partial Pressure : Outport
  Nernest Voltage (V) : Outport  Port=2
  Water Pressure : Outport  Port=3
  wires:
  Air Pressure (atm)/1 -> From Absolute Pressure (atm) To Partial Pressures (atm)/3(Air Pressure (P_air))
  Current Density (i)/1 -> From Absolute Pressure (atm) To Partial Pressures (atm)/1(Current Density (i ))
  From Absolute Pressure (atm) To Partial Pressures (atm)/3(Water Pressure) -> From Partial Pressures (atm) To Nernest Voltage (V)/3(Water Pressure (P_H2O)), Water Pressure/1
  From Absolute Pressure (atm) To Partial Pressures (atm)/2(Oxygen Partial Pressure pp_O2) -> From Partial Pressures (atm) To Nernest Voltage (V)/2(Oxygen Partial Pressure), Oxygen Partial Pressure/1
  From Partial Pressures (atm) To Nernest Voltage (V)/1(Nernest Voltage1) -> Nernest Voltage (V)/1
  Hydrogen Pressure (atm)/1 -> From Absolute Pressure (atm) To Partial Pressures (atm)/2(Hydrogen Pressure (P_H2))
  From Absolute Pressure (atm) To Partial Pressures (atm)/1(Hydrogen Partial Pressure (pp_H2)) -> From Partial Pressures (atm) To Nernest Voltage (V)/1(Hydrogen Partial Pressure)
  Temperature (C)/1 -> From Absolute Pressure (atm) To Partial Pressures (atm)/4(Temperature/C), From Partial Pressures (atm) To Nernest Voltage (V)/4(Temperature/C)

== system Final_System_Model_V10/Full System/Subsystem1/80KW Fuel Cell Stack_1/Load/Current from Load profile of one day ==
  Demux : Demux  Tag=STV Demux  Outputs=2
  FromWs : FromWorkspace  Tag=STV FromWs  VariableName=tuvar  SampleTime=0
      SigBuilderData=|
      | common.afterFinalStr = 'Extrapolate'
      | common.sampleTime = 0
      | dataSet.timeRange = [0 300]
      | dataSet.name = 'Group 1'
      | sbobj.Groups.Name = 'Group 1'
      | sbobj.Groups.Signals(1).Name = 'Signal 1'
      | sbobj.Groups.Signals(1).XData = [0 2.75 2.75 5.75 5.75 10.98 10.98 24 24 24.6 24.6 27.61 27.61 30.61 30.61 33.73 33.73 36.73 48 48 52.19 52.19 55.19 55.19 59.38 59.38 62.38 72 72 84 84 96 96 108 108 120 120 132 132 144 144 146.76 146.76 147.76 147.76 156 156 168 168 175.76 175.76 176.76 176.76 180 180 192 192 204 204 216 216 216.76 216.76 217.76 217.76 228 228 240 240 244.83 244.83 300]
      | sbobj.Groups.Signals(1).YData = [145.4545455 145.4545455 0.01 0.01 145.4545455 145.4545455 0.01 0.01 195.4545455 195.4545455 486.3636364 486.3636364 0.01 0.01 404.5454545 404.5454545 0.01 0.01 0.01 486.3636364 486.3636364 0.01 0.01 486.3636364 486.3636364 0.01 0.01 0.01 463.6363636 463.6363636 0.01 0.01 463.6363636 463.6363636 0.01 0.01 463.6363636 463.6363636 0.01 0.01 463.6363636 463.6363636 0.01 0.01 463.6363636 463.6363636 0.01 0.01 463.6363636 463.6363636 0.01 0.01 463.6363636 463.6363636 0.01 0.01 463.6363636 463.6363636 0.01 0.01 463.6363636 463.6363636 0.01 0.01 463.6363636 463.6363636 0.01 0.01 463.6363636 463.6363636 0.01 0.01]
      | sbobj.Groups.Signals(2).Name = 'Signal 2'
      | sbobj.Groups.Signals(2).XData = [0 300]
      | sbobj.Groups.Signals(2).YData = [243 243]
      | sbobj.Groups.TimeRange = [0 300]
  Signal 1 : Outport  Tag=STV Outport
  Signal 2 : Outport  Tag=STV Outport  Port=2
  wires:
  Demux/2 -> Signal 2/1
  FromWs/1 -> Demux/1
  Demux/1 -> Signal 1/1

== system Final_System_Model_V10/Full System/Electrolysers/260 KW Electrolyzer Stack_1/electrolyser stack/electrolyser cell/(1//T)//(1//T_ref) ==
  In1 : Inport
  In2 : Inport  Port=2
  Constant : Constant
  Divide1 : Product  Inputs=*/
  Divide2 : Product  Inputs=*/
  Out1 : Outport
  wires:
  Divide1/1 -> Divide2/1
  Constant/1 -> Divide1/1
  In2/1 -> Divide2/2
  Divide2/1 -> Out1/1
  In1/1 -> Divide1/2

== system Final_System_Model_V10/Full System/Electrolysers/260 KW Electrolyzer Stack_1/electrolyser stack/electrolyser cell/Eta_B ==
  In1 : Inport
  In2 : Inport  Port=2
  In3 : Inport  Port=3
  In4 : Inport  Port=4
  L_B : Constant  Value=175e-4
  Product : Product  Inputs=*/
  Product1 : Product
  segma_B : Subsystem
  Out1 : Outport
  wires:
  segma_B/1(Out1) -> Product/2
  L_B/1 -> Product/1
  Product1/1 -> Out1/1
  In3/1 -> Product1/2
  Product/1 -> Product1/1
  In2/1 -> segma_B/2(In2)
  In4/1 -> segma_B/3(In4)
  In1/1 -> segma_B/1(In1)

== system Final_System_Model_V10/Full System/Electrolysers/260 KW Electrolyzer Stack_1/electrolyser stack/electrolyser cell/H2 flow rate ==
  In1 : Inport
  In2 : Inport  Port=2
  In3 : Inport  Port=3
  Divide : Product  Inputs=*/
  Multiply : Product
  Out1 : Outport
  wires:
  Multiply/1 -> Divide/1
  In1/1 -> Multiply/1
  In3/1 -> Multiply/2
  In2/1 -> Divide/2
  Divide/1 -> Out1/1

== system Final_System_Model_V10/Full System/Electrolysers/260 KW Electrolyzer Stack_1/electrolyser stack/electrolyser cell/V_0 ==
  In1 : Inport
  Add : Sum  Inputs=+-
  Add1 : Sum  Inputs=+-
  Constant : Constant  Value=8.46e-4
  OCV : Constant  Value=1.229
  Product : Product
  T_ref : Constant  Value=298
  Out1 : Outport
  wires:
  OCV/1 -> Add/1
  Add/1 -> Out1/1
  Product/1 -> Add/2
  T_ref/1 -> Add1/2
  In1/1 -> Add1/1
  Constant/1 -> Product/1
  Add1/1 -> Product/2

== system Final_System_Model_V10/Full System/Electrolysers/260 KW Electrolyzer Stack_1/electrolyser stack/electrolyser cell/eta_a ==
  In1 : Inport
  In2 : Inport  Port=2
  In3 : Inport  Port=3
  In4 : Inport  Port=4
  In5 : Inport  Port=5
  In6 : Inport  Port=6
  B_a : Constant  Value=5
  Divide : Product  Inputs=*/
  Divide1 : Product  Inputs=*/
  Gain : Gain  Gain=0.5
  Multiply : Product
  Multiply1 : Product  Inputs=3
  Multiply2 : Product
  Sin : Trigonometry  Operator=asinh
  m_a : Subsystem
  n_a : Subsystem
  v_a : Constant  Value=3
  Out1 : Outport
  wires:
  n_a/1(Out1) -> Divide1/1
  B_a/1 -> Multiply1/1
  Divide1/1 -> Gain/1
  In1/1 -> n_a/1(In1)
  Sin/1 -> Multiply2/1
  Multiply/1 -> Divide/1
  In6/1 -> Multiply1/3
  Gain/1 -> Sin/1
  Multiply1/1 -> Divide/2
  In3/1 -> n_a/3(In3), m_a/1(In1)
  Multiply2/1 -> Out1/1
  Divide/1 -> Multiply2/2
  v_a/1 -> Multiply1/2
  m_a/1(Out1) -> Divide1/2
  In5/1 -> Multiply/2
  In4/1 -> Multiply/1
  In2/1 -> n_a/2(In2)

== system Final_System_Model_V10/Full System/Electrolysers/260 KW Electrolyzer Stack_1/electrolyser stack/electrolyser cell/eta_c ==
  In1 : Inport
  In2 : Inport  Port=2
  In3 : Inport  Port=3
  In4 : Inport  Port=4
  In5 : Inport  Port=5
  B_c : Constant  Value=5
  Divide : Product  Inputs=*/
  Divide1 : Product  Inputs=*/
  Gain : Gain  Gain=0.5
  Multiply : Product
  Multiply1 : Product  Inputs=3
  Multiply2 : Product
  Sin : Trigonometry  Operator=asinh
  m_c : Subsystem
  n_c : Subsystem
  v_c : Constant  Value=-1
  Out1 : Outport
  wires:
  In1/1 -> n_c/1(In1)
  In2/1 -> Multiply/1, n_c/2(In2)
  Multiply/1 -> Divide/1
  Divide1/1 -> Gain/1
  n_c/1(Out1) -> Divide1/1
  v_c/1 -> Multiply1/3
  In4/1 -> m_c/1(In1), n_c/3(In3)
  B_c/1 -> Multiply1/1
  Multiply1/1 -> Divide/2
  Sin/1 -> Multiply2/1
  m_c/1(Out1) -> Divide1/2
  Divide/1 -> Multiply2/2
  Gain/1 -> Sin/1
  Multiply2/1 -> Out1/1
  In3/1 -> Multiply/2
  In5/1 -> Multiply1/2

== system Final_System_Model_V10/Full System/Electrolysers/93 KW Electrolyzer Stack_2/electrolyser stack/electrolyser cell/(1//T)//(1//T_ref) ==
  In1 : Inport
  In2 : Inport  Port=2
  Constant : Constant
  Divide1 : Product  Inputs=*/
  Divide2 : Product  Inputs=*/
  Out1 : Outport
  wires:
  In1/1 -> Divide1/2
  Divide2/1 -> Out1/1
  In2/1 -> Divide2/2
  Constant/1 -> Divide1/1
  Divide1/1 -> Divide2/1

== system Final_System_Model_V10/Full System/Electrolysers/93 KW Electrolyzer Stack_2/electrolyser stack/electrolyser cell/Eta_B ==
  In1 : Inport
  In2 : Inport  Port=2
  In3 : Inport  Port=3
  In4 : Inport  Port=4
  L_B : Constant  Value=175e-4
  Product : Product  Inputs=*/
  Product1 : Product
  segma_B : Subsystem
  Out1 : Outport
  wires:
  In1/1 -> segma_B/1(In1)
  In4/1 -> segma_B/3(In4)
  In2/1 -> segma_B/2(In2)
  Product/1 -> Product1/1
  In3/1 -> Product1/2
  Product1/1 -> Out1/1
  L_B/1 -> Product/1
  segma_B/1(Out1) -> Product/2

== system Final_System_Model_V10/Full System/Electrolysers/93 KW Electrolyzer Stack_2/electrolyser stack/electrolyser cell/H2 flow rate ==
  In1 : Inport
  In2 : Inport  Port=2
  In3 : Inport  Port=3
  Divide : Product  Inputs=*/
  Multiply : Product
  Out1 : Outport
  wires:
  Divide/1 -> Out1/1
  In2/1 -> Divide/2
  In3/1 -> Multiply/2
  In1/1 -> Multiply/1
  Multiply/1 -> Divide/1

== system Final_System_Model_V10/Full System/Electrolysers/93 KW Electrolyzer Stack_2/electrolyser stack/electrolyser cell/V_0 ==
  In1 : Inport
  Add : Sum  Inputs=+-
  Add1 : Sum  Inputs=+-
  Constant : Constant  Value=8.46e-4
  OCV : Constant  Value=1.229
  Product : Product
  T_ref : Constant  Value=298
  Out1 : Outport
  wires:
  Add1/1 -> Product/2
  Constant/1 -> Product/1
  In1/1 -> Add1/1
  T_ref/1 -> Add1/2
  Product/1 -> Add/2
  Add/1 -> Out1/1
  OCV/1 -> Add/1

== system Final_System_Model_V10/Full System/Electrolysers/93 KW Electrolyzer Stack_2/electrolyser stack/electrolyser cell/eta_a ==
  In1 : Inport
  In2 : Inport  Port=2
  In3 : Inport  Port=3
  In4 : Inport  Port=4
  In5 : Inport  Port=5
  In6 : Inport  Port=6
  B_a : Constant  Value=5
  Divide : Product  Inputs=*/
  Divide1 : Product  Inputs=*/
  Gain : Gain  Gain=0.5
  Multiply : Product
  Multiply1 : Product  Inputs=3
  Multiply2 : Product
  Sin : Trigonometry  Operator=asinh
  m_a : Subsystem
  n_a : Subsystem
  v_a : Constant  Value=3
  Out1 : Outport
  wires:
  In2/1 -> n_a/2(In2)
  In4/1 -> Multiply/1
  In5/1 -> Multiply/2
  m_a/1(Out1) -> Divide1/2
  v_a/1 -> Multiply1/2
  Divide/1 -> Multiply2/2
  Multiply2/1 -> Out1/1
  In3/1 -> m_a/1(In1), n_a/3(In3)
  Multiply1/1 -> Divide/2
  Gain/1 -> Sin/1
  In6/1 -> Multiply1/3
  Multiply/1 -> Divide/1
  Sin/1 -> Multiply2/1
  In1/1 -> n_a/1(In1)
  Divide1/1 -> Gain/1
  B_a/1 -> Multiply1/1
  n_a/1(Out1) -> Divide1/1

== system Final_System_Model_V10/Full System/Electrolysers/93 KW Electrolyzer Stack_2/electrolyser stack/electrolyser cell/eta_c ==
  In1 : Inport
  In2 : Inport  Port=2
  In3 : Inport  Port=3
  In4 : Inport  Port=4
  In5 : Inport  Port=5
  B_c : Constant  Value=5
  Divide : Product  Inputs=*/
  Divide1 : Product  Inputs=*/
  Gain : Gain  Gain=0.5
  Multiply : Product
  Multiply1 : Product  Inputs=3
  Multiply2 : Product
  Sin : Trigonometry  Operator=asinh
  m_c : Subsystem
  n_c : Subsystem
  v_c : Constant  Value=-1
  Out1 : Outport
  wires:
  In5/1 -> Multiply1/2
  In3/1 -> Multiply/2
  Multiply2/1 -> Out1/1
  Gain/1 -> Sin/1
  Divide/1 -> Multiply2/2
  m_c/1(Out1) -> Divide1/2
  Sin/1 -> Multiply2/1
  Multiply1/1 -> Divide/2
  B_c/1 -> Multiply1/1
  In4/1 -> n_c/3(In3), m_c/1(In1)
  v_c/1 -> Multiply1/3
  n_c/1(Out1) -> Divide1/1
  Divide1/1 -> Gain/1
  Multiply/1 -> Divide/1
  In2/1 -> n_c/2(In2), Multiply/1
  In1/1 -> n_c/1(In1)

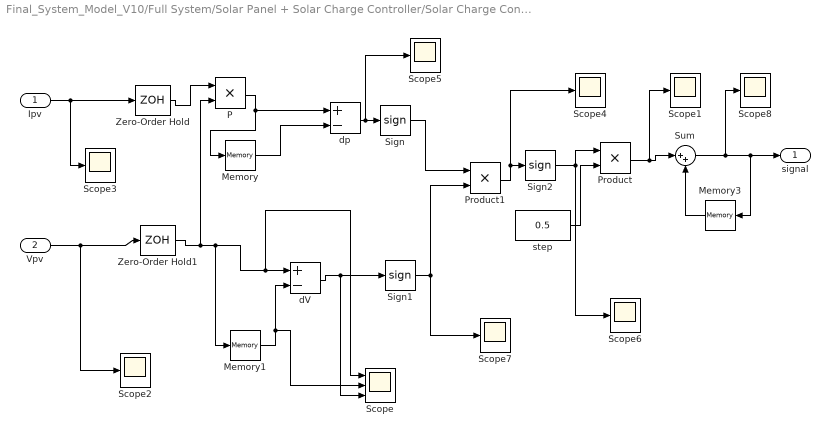
== system Final_System_Model_V10/Full System/Solar Panel + Solar Charge Controller/Solar Charge Controller MPPT it is a device which track a point which has the max power/MPPT /P&O /P & O ==
  Ipv : Inport
  Vpv : Inport  Port=2
  Memory : Memory  InheritSampleTime=on
  Memory1 : Memory  InheritSampleTime=on
  Memory3 : Memory  InheritSampleTime=on
  P : Product  RndMeth=Zero
  Product : Product  RndMeth=Zero
  Product1 : Product  RndMeth=Zero
  Scope : Scope  NumInputPorts=3
  Scope{1..8} (8 alike) : Scope
  Sign : Signum
  Sign1 : Signum
  Sign2 : Signum
  Sum : Sum  Inputs=|++
  Zero-Order Hold : ZeroOrderHold  SampleTime=0.002
  Zero-Order Hold1 : ZeroOrderHold  SampleTime=0.002
  dV : Sum  Inputs=+-
  dp : Sum  Inputs=+-
  step : Constant  Value=0.5
  signal : Outport
  wires:
  Memory1/1 -> dV/2, Scope/2
  Memory/1 -> dp/2
  Vpv/1 -> Zero-Order Hold1/1, Scope2/1
  dV/1 -> Sign1/1, Scope/3
  step/1 -> Product/2
  Product/1 -> Sum/1, Scope1/1
  Sign/1 -> Product1/1
  Sign1/1 -> Product1/2, Scope7/1
  Product1/1 -> Sign2/1, Scope4/1
  Ipv/1 -> Zero-Order Hold/1, Scope3/1
  Zero-Order Hold1/1 -> P/2, dV/1, Scope/1, Memory1/1
  Zero-Order Hold/1 -> P/1
  P/1 -> Memory/1, dp/1
  dp/1 -> Sign/1, Scope5/1
  Sign2/1 -> Product/1, Scope6/1
  Sum/1 -> Memory3/1, signal/1, Scope8/1
  Memory3/1 -> Sum/2

== system Final_System_Model_V10/Full System/Solar Panel + Solar Charge Controller/Solar Charge Controller MPPT it is a device which track a point which has the max power/MPPT /P&O /Subsystem1 ==
  In1 : Inport
  Compare To Zero : simulink/Logic and Bit Operations/Compare To Zero  relop=<=  OutDataTypeStr=boolean
  Repeating Sequence : simulink/Sources/Repeating Sequence  rep_seq_t=[0 0.1e-3]  rep_seq_y=[0 1]
  Subtract : Sum  Inputs=+-
  Out1 : Outport
  wires:
  Subtract/1 -> Compare To Zero/1
  Repeating Sequence/1 -> Subtract/2
  In1/1 -> Subtract/1
  Compare To Zero/1 -> Out1/1
